simulink model "rls_param_est_2019_01_12"  (R2020a)
settings: Solver=VariableStepAuto  StartTime=0.0  StopTime=simlength  MaxStep=Ts  RelTol=Ts
undefined symbols (not defined in the file or in its folder): iniP11, iniP12, iniP13, iniP14, iniP21, iniP22, iniP23, iniP24, iniP31, iniP32, iniP33, iniP34, iniP41, iniP42, iniP43, iniP44, lambda, simlength, Tc, Tcontrol, Ts
libraries: cstblocks x5, simulink x1
settings Model: SimulationMode=accelerator  Creator=ltnbda  LastModifiedBy=dbagn
settings DataIOCC: ReturnWorkspaceOutputs=off
settings DebuggingCC: ArithmeticOperatorsInVariantConditions=warning
settings SFSimCC: CustomCodeUndefinedFunction=UseInterfaceOnly

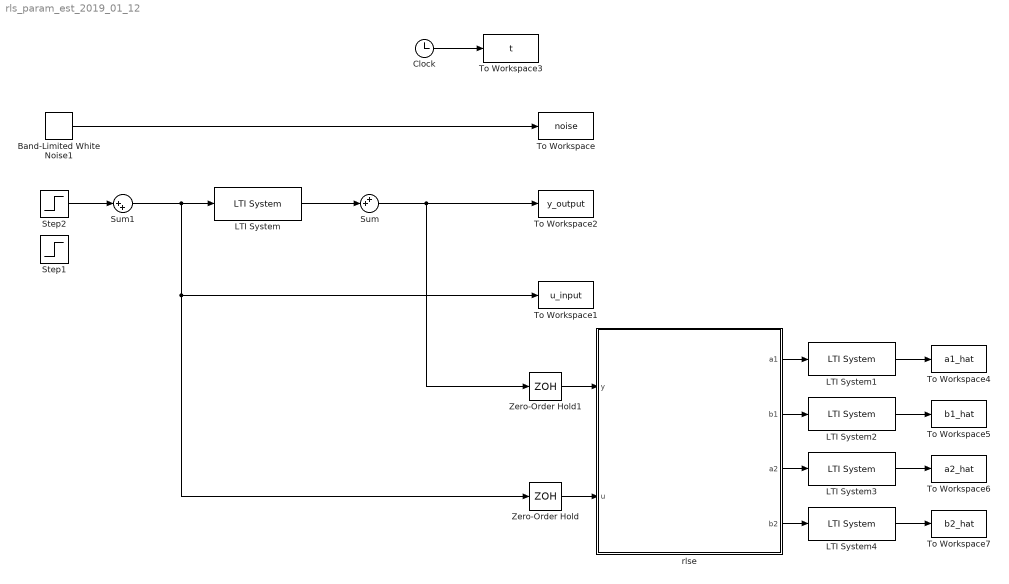
== system rls_param_est_2019_01_12 ==
  Band-Limited White Noise1 : simulink/Sources/Band-Limited White Noise  Cov=[1e-12]  Ts=Ts  seed=[0]
  Clock : Clock
  LTI System : cstblocks/LTI System  sys=sysIc  IC=[]
  LTI System{1..4} (4 alike) : cstblocks/LTI System  sys=filterd  IC=[]
  Step1 : Step  Time=simlength/2  After=0.5  SampleTime=Tcontrol
  Step2 : Step  Time=0.05  After=0.5  SampleTime=Tcontrol
  Sum : Sum  Inputs=++|
  Sum1 : Sum  Inputs=|++
  To Workspace : ToWorkspace  VariableName=noise  SampleTime=Tc
      settings: MaxDataPoints=Nc
  To Workspace1 : ToWorkspace  VariableName=u_input  SampleTime=Tc
      settings: MaxDataPoints=Nc
  To Workspace2 : ToWorkspace  VariableName=y_output  SampleTime=Tc
      settings: MaxDataPoints=Nc
  To Workspace3 : ToWorkspace  VariableName=t  SampleTime=Tc
      settings: MaxDataPoints=Nc
  To Workspace4 : ToWorkspace  VariableName=a1_hat  SampleTime=Tc
      settings: MaxDataPoints=Nc
  To Workspace5 : ToWorkspace  VariableName=b1_hat  SampleTime=Tc
      settings: MaxDataPoints=Nc
  To Workspace6 : ToWorkspace  VariableName=a2_hat  SampleTime=Tc
      settings: MaxDataPoints=Nc
  To Workspace7 : ToWorkspace  VariableName=b2_hat  SampleTime=Tc
      settings: MaxDataPoints=Nc
  Zero-Order Hold : ZeroOrderHold  SampleTime=Tcontrol
  Zero-Order Hold1 : ZeroOrderHold  SampleTime=Tcontrol
  rlse : Subsystem
  wires:
  LTI System/1 -> Sum/2
  Zero-Order Hold/1 -> rlse/2(u)
  Zero-Order Hold1/1 -> rlse/1(y)
  Sum/1 -> To Workspace2/1, Zero-Order Hold1/1
  Sum1/1 -> Zero-Order Hold/1, To Workspace1/1, LTI System/1
  Band-Limited White Noise1/1 -> To Workspace/1
  Clock/1 -> To Workspace3/1
  rlse/1(a1) -> LTI System1/1
  rlse/3(a2) -> LTI System3/1
  rlse/4(b2) -> LTI System4/1
  rlse/2(b1) -> LTI System2/1
  LTI System1/1 -> To Workspace4/1
  LTI System2/1 -> To Workspace5/1
  LTI System3/1 -> To Workspace6/1
  LTI System4/1 -> To Workspace7/1
  Step2/1 -> Sum1/1

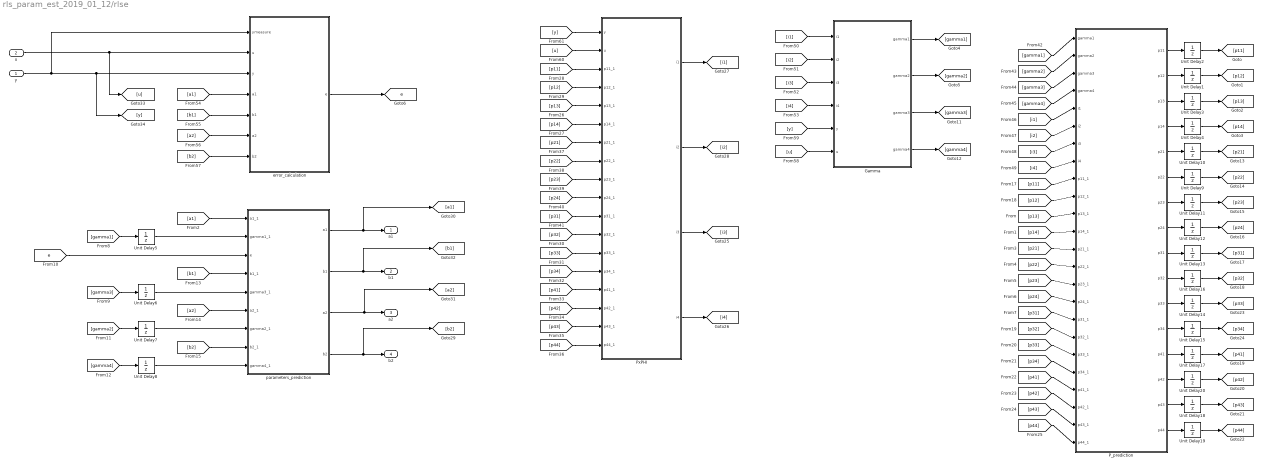
== system rls_param_est_2019_01_12/rlse ==
  y : Inport
  u : Inport  Port=2
  Gamma : Subsystem
  P_prediction : Subsystem
  PxPHI : Subsystem
  Unit Delay1 : UnitDelay  InitialCondition=iniP12  SampleTime=Tcontrol  HasFrameUpgradeWarning=on
  Unit Delay10 : UnitDelay  InitialCondition=iniP21  SampleTime=Tcontrol  HasFrameUpgradeWarning=on
  Unit Delay11 : UnitDelay  InitialCondition=iniP23  SampleTime=Tcontrol  HasFrameUpgradeWarning=on
  Unit Delay12 : UnitDelay  InitialCondition=iniP24  SampleTime=Tcontrol  HasFrameUpgradeWarning=on
  Unit Delay13 : UnitDelay  InitialCondition=iniP31  SampleTime=Tcontrol  HasFrameUpgradeWarning=on
  Unit Delay14 : UnitDelay  InitialCondition=iniP33  SampleTime=Tcontrol  HasFrameUpgradeWarning=on
  Unit Delay15 : UnitDelay  InitialCondition=iniP34  SampleTime=Tcontrol  HasFrameUpgradeWarning=on
  Unit Delay16 : UnitDelay  InitialCondition=iniP32  SampleTime=Tcontrol  HasFrameUpgradeWarning=on
  Unit Delay17 : UnitDelay  InitialCondition=iniP41  SampleTime=Tcontrol  HasFrameUpgradeWarning=on
  Unit Delay18 : UnitDelay  InitialCondition=iniP43  SampleTime=Tcontrol  HasFrameUpgradeWarning=on
  Unit Delay19 : UnitDelay  InitialCondition=iniP44  SampleTime=Tcontrol  HasFrameUpgradeWarning=on
  Unit Delay2 : UnitDelay  InitialCondition=iniP11  SampleTime=Tcontrol  HasFrameUpgradeWarning=on
  Unit Delay20 : UnitDelay  InitialCondition=iniP42  SampleTime=Tcontrol  HasFrameUpgradeWarning=on
  Unit Delay3 : UnitDelay  InitialCondition=iniP13  SampleTime=Tcontrol  HasFrameUpgradeWarning=on
  Unit Delay4 : UnitDelay  InitialCondition=iniP14  SampleTime=Tcontrol  HasFrameUpgradeWarning=on
  Unit Delay{5..8} (4 alike) : UnitDelay  SampleTime=Tcontrol  HasFrameUpgradeWarning=on
  Unit Delay9 : UnitDelay  InitialCondition=iniP22  SampleTime=Tcontrol  HasFrameUpgradeWarning=on
  error_calculation : Subsystem
  parameters_prediction : Subsystem
  a1 : Outport  VectorParamsAs1DForOutWhenUnconnected=off
  b1 : Outport  Port=2  VectorParamsAs1DForOutWhenUnconnected=off
  a2 : Outport  Port=3  VectorParamsAs1DForOutWhenUnconnected=off
  b2 : Outport  Port=4  VectorParamsAs1DForOutWhenUnconnected=off
  tag scope: e=global
  wires:
  u/1 -> [u], error_calculation/2(u)
  Unit Delay2/1 -> [p11]
  [gamma1] -> Unit Delay5/1
  [gamma3] -> Unit Delay6/1
  Unit Delay1/1 -> [p12]
  Unit Delay3/1 -> [p13]
  Unit Delay4/1 -> [p14]
  Unit Delay5/1 -> parameters_prediction/2(gamma1_1)
  Unit Delay6/1 -> parameters_prediction/5(gamma3_1)
  error_calculation/1(e) -> [e]
  [e] -> parameters_prediction/3(e)
  [gamma4] -> Unit Delay8/1
  [gamma2] -> Unit Delay7/1
  Unit Delay7/1 -> parameters_prediction/7(gamma2_1)
  Unit Delay8/1 -> parameters_prediction/9(gamma4_1)
  Gamma/1(gamma1) -> [gamma1]
  Gamma/2(gamma2) -> [gamma2]
  Gamma/3(gamma3) -> [gamma3]
  Gamma/4(gamma4) -> [gamma4]
  P_prediction/1(p11) -> Unit Delay2/1
  P_prediction/2(p12) -> Unit Delay1/1
  P_prediction/3(p13) -> Unit Delay3/1
  P_prediction/4(p14) -> Unit Delay4/1
  P_prediction/8(p24) -> Unit Delay12/1
  P_prediction/7(p23) -> Unit Delay11/1
  P_prediction/6(p22) -> Unit Delay9/1
  P_prediction/5(p21) -> Unit Delay10/1
  Unit Delay12/1 -> [p24]
  Unit Delay11/1 -> [p23]
  Unit Delay9/1 -> [p22]
  Unit Delay10/1 -> [p21]
  Unit Delay17/1 -> [p41]
  Unit Delay20/1 -> [p42]
  Unit Delay18/1 -> [p43]
  Unit Delay19/1 -> [p44]
  P_prediction/13(p41) -> Unit Delay17/1
  P_prediction/14(p42) -> Unit Delay20/1
  P_prediction/15(p43) -> Unit Delay18/1
  P_prediction/16(p44) -> Unit Delay19/1
  P_prediction/12(p34) -> Unit Delay15/1
  P_prediction/11(p33) -> Unit Delay14/1
  P_prediction/10(p32) -> Unit Delay16/1
  P_prediction/9(p31) -> Unit Delay13/1
  Unit Delay15/1 -> [p34]
  Unit Delay14/1 -> [p33]
  Unit Delay16/1 -> [p32]
  Unit Delay13/1 -> [p31]
  [p11] -> P_prediction/9(p11_1)
  [p13] -> P_prediction/11(p13_1)
  [p12] -> P_prediction/10(p12_1)
  [p14] -> P_prediction/12(p14_1)
  [p21] -> P_prediction/13(p21_1)
  [p22] -> P_prediction/14(p22_1)
  [p23] -> P_prediction/15(p23_1)
  [p24] -> P_prediction/16(p24_1)
  [p31] -> P_prediction/17(p31_1)
  [p32] -> P_prediction/18(p32_1)
  [p33] -> P_prediction/19(p33_1)
  [p34] -> P_prediction/20(p34_1)
  [p41] -> P_prediction/21(p41_1)
  [p42] -> P_prediction/22(p42_1)
  [p43] -> P_prediction/23(p43_1)
  [p44] -> P_prediction/24(p44_1)
  [p44] -> PxPHI/18(p44_1)
  [p43] -> PxPHI/17(p43_1)
  [p42] -> PxPHI/16(p42_1)
  [p41] -> PxPHI/15(p41_1)
  [p34] -> PxPHI/14(p34_1)
  [p33] -> PxPHI/13(p33_1)
  [p32] -> PxPHI/12(p32_1)
  [p31] -> PxPHI/11(p31_1)
  [p24] -> PxPHI/10(p24_1)
  [p23] -> PxPHI/9(p23_1)
  [p22] -> PxPHI/8(p22_1)
  [p21] -> PxPHI/7(p21_1)
  [p14] -> PxPHI/6(p14_1)
  [p12] -> PxPHI/4(p12_1)
  [p13] -> PxPHI/5(p13_1)
  [p11] -> PxPHI/3(p11_1)
  [gamma1] -> P_prediction/1(gamma1)
  [gamma2] -> P_prediction/2(gamma2)
  [gamma3] -> P_prediction/3(gamma3)
  [gamma4] -> P_prediction/4(gamma4)
  PxPHI/4(i4) -> [i4]
  PxPHI/3(i3) -> [i3]
  PxPHI/2(i2) -> [i2]
  PxPHI/1(i1) -> [i1]
  [i1] -> P_prediction/5(i1)
  [i2] -> P_prediction/6(i2)
  [i3] -> P_prediction/7(i3)
  [i4] -> P_prediction/8(i4)
  [i2] -> Gamma/2(i2)
  [i1] -> Gamma/1(i1)
  [i3] -> Gamma/3(i3)
  [i4] -> Gamma/4(i4)
  parameters_prediction/4(b2) -> [b2], b2/1
  parameters_prediction/3(a2) -> [a2], a2/1
  parameters_prediction/2(b1) -> [b1], b1/1
  parameters_prediction/1(a1) -> [a1], a1/1
  [a1] -> error_calculation/4(a1)
  [b1] -> error_calculation/5(b1)
  [a2] -> error_calculation/6(a2)
  [b2] -> error_calculation/7(b2)
  [u] -> Gamma/6(u)
  [y] -> Gamma/5(y)
  [y] -> PxPHI/1(y)
  [u] -> PxPHI/2(u)
  y/1 -> [y], error_calculation/3(y), error_calculation/1(ymeasure)
  [a1] -> parameters_prediction/1(a1_1)
  [b1] -> parameters_prediction/4(b1_1)
  [a2] -> parameters_prediction/6(a2_1)
  [b2] -> parameters_prediction/8(b2_1)

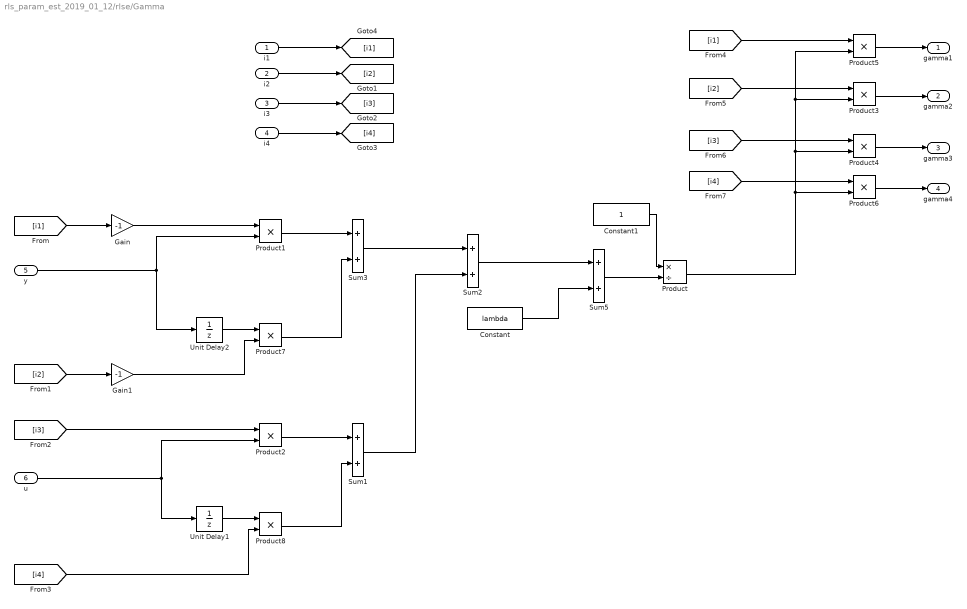
== system rls_param_est_2019_01_12/rlse/Gamma ==
  i1 : Inport
  i2 : Inport  Port=2
  i3 : Inport  Port=3
  i4 : Inport  Port=4
  y : Inport  Port=5
  u : Inport  Port=6
  Constant : Constant  Value=lambda
  Constant1 : Constant
  Gain : Gain  Gain=-1
  Gain1 : Gain  Gain=-1
  Product : Product  Inputs=*/
  Product{1..8} (8 alike) : Product
  Sum{1..3,5} (4 alike) : Sum
  Unit Delay1 : UnitDelay  SampleTime=Tcontrol  HasFrameUpgradeWarning=on
  Unit Delay2 : UnitDelay  SampleTime=Tcontrol  HasFrameUpgradeWarning=on
  gamma1 : Outport  VectorParamsAs1DForOutWhenUnconnected=off
  gamma2 : Outport  Port=2  VectorParamsAs1DForOutWhenUnconnected=off
  gamma3 : Outport  Port=3  VectorParamsAs1DForOutWhenUnconnected=off
  gamma4 : Outport  Port=4  VectorParamsAs1DForOutWhenUnconnected=off
  wires:
  u/1 -> Product2/2, Unit Delay1/1
  Gain/1 -> Product1/1
  y/1 -> Product1/2, Unit Delay2/1
  Constant1/1 -> Product/1
  Product3/1 -> gamma2/1
  Product5/1 -> gamma1/1
  Product4/1 -> gamma3/1
  Product6/1 -> gamma4/1
  Product1/1 -> Sum3/1
  Unit Delay2/1 -> Product7/1
  Gain1/1 -> Product7/2
  Product7/1 -> Sum3/2
  Product2/1 -> Sum1/1
  Product8/1 -> Sum1/2
  Sum3/1 -> Sum2/1
  Sum1/1 -> Sum2/2
  Product/1 -> Product6/2, Product4/2, Product3/2, Product5/2
  Sum2/1 -> Sum5/1
  Constant/1 -> Sum5/2
  Sum5/1 -> Product/2
  i1/1 -> [i1]
  i2/1 -> [i2]
  i3/1 -> [i3]
  i4/1 -> [i4]
  [i1] -> Gain/1
  [i2] -> Gain1/1
  [i3] -> Product2/1
  [i4] -> Product8/2
  [i1] -> Product5/1
  [i2] -> Product3/1
  [i3] -> Product4/1
  [i4] -> Product6/1
  Unit Delay1/1 -> Product8/1

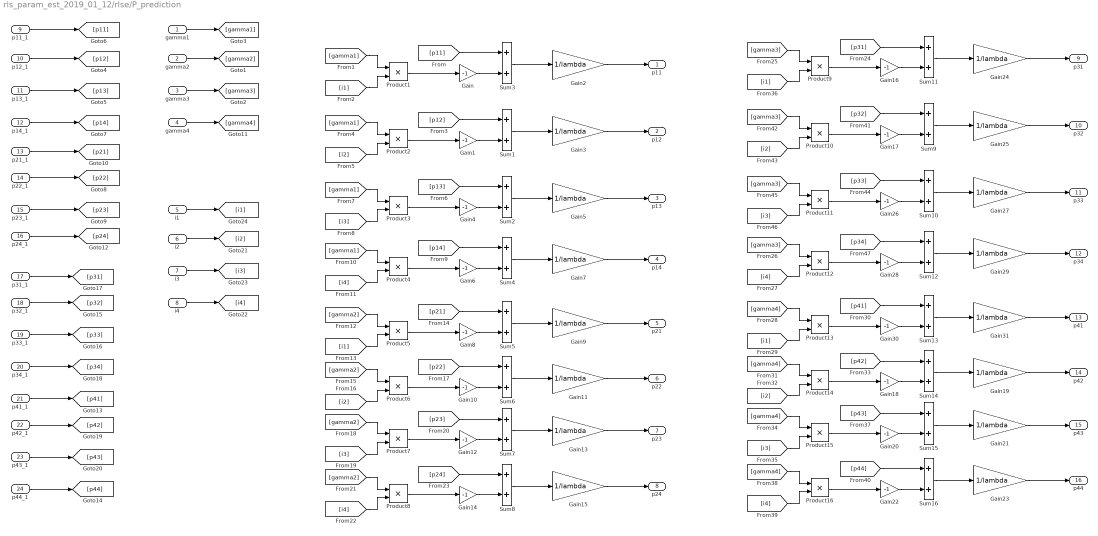
== system rls_param_est_2019_01_12/rlse/P_prediction ==
  gamma1 : Inport
  gamma2 : Inport  Port=2
  gamma3 : Inport  Port=3
  gamma4 : Inport  Port=4
  i1 : Inport  Port=5
  i2 : Inport  Port=6
  i3 : Inport  Port=7
  i4 : Inport  Port=8
  p11_1 : Inport  Port=9
  p12_1 : Inport  Port=10
  p13_1 : Inport  Port=11
  p14_1 : Inport  Port=12
  p21_1 : Inport  Port=13
  p22_1 : Inport  Port=14
  p23_1 : Inport  Port=15
  p24_1 : Inport  Port=16
  p31_1 : Inport  Port=17
  p32_1 : Inport  Port=18
  p33_1 : Inport  Port=19
  p34_1 : Inport  Port=20
  p41_1 : Inport  Port=21
  p42_1 : Inport  Port=22
  p43_1 : Inport  Port=23
  p44_1 : Inport  Port=24
  Gain{,1,4,6,8,10,12,14,16..18,20,22,26,28,30} (16 alike) : Gain  Gain=-1
  Gain{2..3,5,7,9,11,13,15,19,21,23..25,27,29,31} (16 alike) : Gain  Gain=1/lambda
  Product{1..16} (16 alike) : Product
  Sum{1..16} (16 alike) : Sum
  p11 : Outport  VectorParamsAs1DForOutWhenUnconnected=off
  p12 : Outport  Port=2  VectorParamsAs1DForOutWhenUnconnected=off
  p13 : Outport  Port=3  VectorParamsAs1DForOutWhenUnconnected=off
  p14 : Outport  Port=4  VectorParamsAs1DForOutWhenUnconnected=off
  p21 : Outport  Port=5  VectorParamsAs1DForOutWhenUnconnected=off
  p22 : Outport  Port=6  VectorParamsAs1DForOutWhenUnconnected=off
  p23 : Outport  Port=7  VectorParamsAs1DForOutWhenUnconnected=off
  p24 : Outport  Port=8  VectorParamsAs1DForOutWhenUnconnected=off
  p31 : Outport  Port=9  VectorParamsAs1DForOutWhenUnconnected=off
  p32 : Outport  Port=10  VectorParamsAs1DForOutWhenUnconnected=off
  p33 : Outport  Port=11  VectorParamsAs1DForOutWhenUnconnected=off
  p34 : Outport  Port=12  VectorParamsAs1DForOutWhenUnconnected=off
  p41 : Outport  Port=13  VectorParamsAs1DForOutWhenUnconnected=off
  p42 : Outport  Port=14  VectorParamsAs1DForOutWhenUnconnected=off
  p43 : Outport  Port=15  VectorParamsAs1DForOutWhenUnconnected=off
  p44 : Outport  Port=16  VectorParamsAs1DForOutWhenUnconnected=off
  wires:
  p11_1/1 -> [p11]
  p12_1/1 -> [p12]
  p13_1/1 -> [p13]
  p14_1/1 -> [p14]
  p21_1/1 -> [p21]
  p22_1/1 -> [p22]
  p23_1/1 -> [p23]
  p24_1/1 -> [p24]
  p31_1/1 -> [p31]
  p32_1/1 -> [p32]
  p33_1/1 -> [p33]
  p34_1/1 -> [p34]
  p41_1/1 -> [p41]
  p42_1/1 -> [p42]
  p43_1/1 -> [p43]
  p44_1/1 -> [p44]
  gamma1/1 -> [gamma1]
  gamma3/1 -> [gamma3]
  gamma2/1 -> [gamma2]
  gamma4/1 -> [gamma4]
  i4/1 -> [i4]
  i2/1 -> [i2]
  i3/1 -> [i3]
  i1/1 -> [i1]
  [p11] -> Sum3/1
  Gain/1 -> Sum3/2
  Product1/1 -> Gain/1
  [gamma1] -> Product1/1
  [i1] -> Product1/2
  Sum3/1 -> Gain2/1
  Gain2/1 -> p11/1
  Sum1/1 -> Gain3/1
  [i2] -> Product2/2
  [gamma1] -> Product2/1
  Product2/1 -> Gain1/1
  Gain1/1 -> Sum1/2
  [p12] -> Sum1/1
  Gain3/1 -> p12/1
  Gain5/1 -> p13/1
  [p13] -> Sum2/1
  Gain4/1 -> Sum2/2
  Product3/1 -> Gain4/1
  [gamma1] -> Product3/1
  [i3] -> Product3/2
  Sum2/1 -> Gain5/1
  Sum4/1 -> Gain7/1
  [i4] -> Product4/2
  [gamma1] -> Product4/1
  Product4/1 -> Gain6/1
  Gain6/1 -> Sum4/2
  [p14] -> Sum4/1
  Gain7/1 -> p14/1
  Gain9/1 -> p21/1
  [p21] -> Sum5/1
  Gain8/1 -> Sum5/2
  Product5/1 -> Gain8/1
  [gamma2] -> Product5/1
  [i1] -> Product5/2
  Sum5/1 -> Gain9/1
  Sum6/1 -> Gain11/1
  [i2] -> Product6/2
  [gamma2] -> Product6/1
  Product6/1 -> Gain10/1
  Gain10/1 -> Sum6/2
  [p22] -> Sum6/1
  Gain11/1 -> p22/1
  Gain13/1 -> p23/1
  [p23] -> Sum7/1
  Gain12/1 -> Sum7/2
  Product7/1 -> Gain12/1
  [gamma2] -> Product7/1
  [i3] -> Product7/2
  Sum7/1 -> Gain13/1
  Sum8/1 -> Gain15/1
  [i4] -> Product8/2
  [gamma2] -> Product8/1
  Product8/1 -> Gain14/1
  Gain14/1 -> Sum8/2
  [p24] -> Sum8/1
  Gain15/1 -> p24/1
  Gain23/1 -> p44/1
  [p44] -> Sum16/1
  Gain22/1 -> Sum16/2
  Product16/1 -> Gain22/1
  [gamma4] -> Product16/1
  [i4] -> Product16/2
  Sum16/1 -> Gain23/1
  Sum15/1 -> Gain21/1
  [i3] -> Product15/2
  [gamma4] -> Product15/1
  Product15/1 -> Gain20/1
  Gain20/1 -> Sum15/2
  [p43] -> Sum15/1
  Gain21/1 -> p43/1
  Gain19/1 -> p42/1
  [p42] -> Sum14/1
  Gain18/1 -> Sum14/2
  Product14/1 -> Gain18/1
  [gamma4] -> Product14/1
  [i2] -> Product14/2
  Sum14/1 -> Gain19/1
  Sum13/1 -> Gain31/1
  [i1] -> Product13/2
  [gamma4] -> Product13/1
  Product13/1 -> Gain30/1
  Gain30/1 -> Sum13/2
  [p41] -> Sum13/1
  Gain31/1 -> p41/1
  Gain29/1 -> p34/1
  [p34] -> Sum12/1
  Gain28/1 -> Sum12/2
  Product12/1 -> Gain28/1
  [gamma3] -> Product12/1
  [i4] -> Product12/2
  Sum12/1 -> Gain29/1
  Sum10/1 -> Gain27/1
  [i3] -> Product11/2
  [gamma3] -> Product11/1
  Product11/1 -> Gain26/1
  Gain26/1 -> Sum10/2
  [p33] -> Sum10/1
  Gain27/1 -> p33/1
  Gain25/1 -> p32/1
  [p32] -> Sum9/1
  Gain17/1 -> Sum9/2
  Product10/1 -> Gain17/1
  [gamma3] -> Product10/1
  [i2] -> Product10/2
  Sum9/1 -> Gain25/1
  Gain24/1 -> p31/1
  Sum11/1 -> Gain24/1
  [i1] -> Product9/2
  [gamma3] -> Product9/1
  Product9/1 -> Gain16/1
  Gain16/1 -> Sum11/2
  [p31] -> Sum11/1

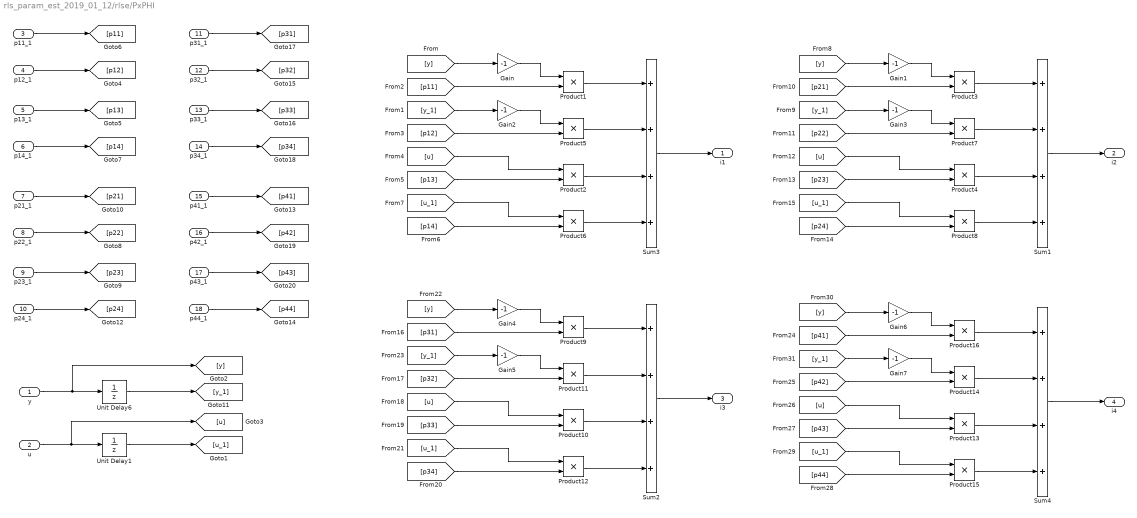
== system rls_param_est_2019_01_12/rlse/PxPHI ==
  y : Inport
  u : Inport  Port=2
  p11_1 : Inport  Port=3
  p12_1 : Inport  Port=4
  p13_1 : Inport  Port=5
  p14_1 : Inport  Port=6
  p21_1 : Inport  Port=7
  p22_1 : Inport  Port=8
  p23_1 : Inport  Port=9
  p24_1 : Inport  Port=10
  p31_1 : Inport  Port=11
  p32_1 : Inport  Port=12
  p33_1 : Inport  Port=13
  p34_1 : Inport  Port=14
  p41_1 : Inport  Port=15
  p42_1 : Inport  Port=16
  p43_1 : Inport  Port=17
  p44_1 : Inport  Port=18
  Gain{,1..7} (8 alike) : Gain  Gain=-1
  Product{1..16} (16 alike) : Product
  Sum{1..4} (4 alike) : Sum  Inputs=++++
  Unit Delay1 : UnitDelay  SampleTime=Tcontrol  HasFrameUpgradeWarning=on
  Unit Delay6 : UnitDelay  SampleTime=Tcontrol  HasFrameUpgradeWarning=on
  i1 : Outport  VectorParamsAs1DForOutWhenUnconnected=off
  i2 : Outport  Port=2  VectorParamsAs1DForOutWhenUnconnected=off
  i3 : Outport  Port=3  VectorParamsAs1DForOutWhenUnconnected=off
  i4 : Outport  Port=4  VectorParamsAs1DForOutWhenUnconnected=off
  wires:
  Sum3/1 -> i1/1
  Product1/1 -> Sum3/1
  Unit Delay6/1 -> [y_1]
  y/1 -> [y], Unit Delay6/1
  u/1 -> [u], Unit Delay1/1
  Unit Delay1/1 -> [u_1]
  p12_1/1 -> [p12]
  p13_1/1 -> [p13]
  p11_1/1 -> [p11]
  p14_1/1 -> [p14]
  p22_1/1 -> [p22]
  p21_1/1 -> [p21]
  p23_1/1 -> [p23]
  p24_1/1 -> [p24]
  p31_1/1 -> [p31]
  p32_1/1 -> [p32]
  p33_1/1 -> [p33]
  p34_1/1 -> [p34]
  p41_1/1 -> [p41]
  p42_1/1 -> [p42]
  p43_1/1 -> [p43]
  p44_1/1 -> [p44]
  Gain/1 -> Product1/1
  Gain2/1 -> Product5/1
  Product5/1 -> Sum3/2
  Product2/1 -> Sum3/3
  Product6/1 -> Sum3/4
  [y] -> Gain/1
  [y_1] -> Gain2/1
  [p11] -> Product1/2
  [p12] -> Product5/2
  [u] -> Product2/1
  [p13] -> Product2/2
  [p14] -> Product6/2
  [u_1] -> Product6/1
  [u_1] -> Product8/1
  [p24] -> Product8/2
  [p23] -> Product4/2
  [u] -> Product4/1
  [p22] -> Product7/2
  [p21] -> Product3/2
  [y_1] -> Gain3/1
  [y] -> Gain1/1
  Product8/1 -> Sum1/4
  Product4/1 -> Sum1/3
  Product7/1 -> Sum1/2
  Gain3/1 -> Product7/1
  Gain1/1 -> Product3/1
  Product3/1 -> Sum1/1
  Sum1/1 -> i2/1
  Sum2/1 -> i3/1
  Product9/1 -> Sum2/1
  Gain4/1 -> Product9/1
  Gain5/1 -> Product11/1
  Product11/1 -> Sum2/2
  Product10/1 -> Sum2/3
  Product12/1 -> Sum2/4
  [y] -> Gain4/1
  [y_1] -> Gain5/1
  [p31] -> Product9/2
  [p32] -> Product11/2
  [u] -> Product10/1
  [p33] -> Product10/2
  [p34] -> Product12/2
  [u_1] -> Product12/1
  [u_1] -> Product15/1
  [p44] -> Product15/2
  [p43] -> Product13/2
  [u] -> Product13/1
  [p42] -> Product14/2
  [p41] -> Product16/2
  [y_1] -> Gain7/1
  [y] -> Gain6/1
  Product15/1 -> Sum4/4
  Product13/1 -> Sum4/3
  Product14/1 -> Sum4/2
  Gain7/1 -> Product14/1
  Gain6/1 -> Product16/1
  Product16/1 -> Sum4/1
  Sum4/1 -> i4/1

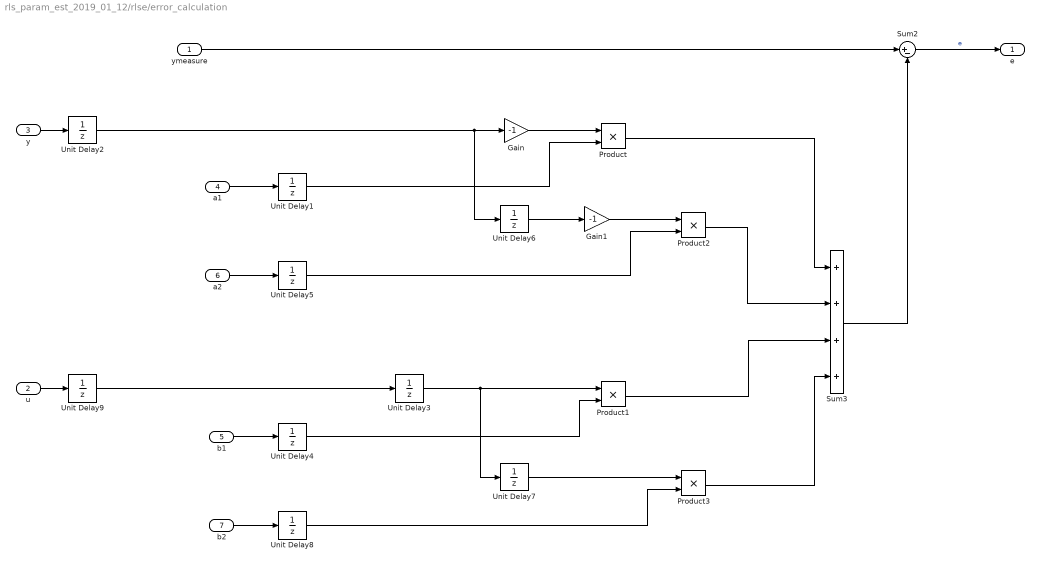
== system rls_param_est_2019_01_12/rlse/error_calculation ==
  ymeasure : Inport
  u : Inport  Port=2
  y : Inport  Port=3
  a1 : Inport  Port=4
  b1 : Inport  Port=5
  a2 : Inport  Port=6
  b2 : Inport  Port=7
  Gain : Gain  Gain=-1
  Gain1 : Gain  Gain=-1
  Product{,1..3} (4 alike) : Product
  Sum2 : Sum  Inputs=|+-
  Sum3 : Sum  Inputs=++++
  Unit Delay{1..9} (9 alike) : UnitDelay  SampleTime=Tcontrol  HasFrameUpgradeWarning=on
  e : Outport  VectorParamsAs1DForOutWhenUnconnected=off
  wires:
  Gain/1 -> Product/1
  Sum3/1 -> Sum2/2
  Sum2/1 -> e/1  "e"
  a1/1 -> Unit Delay1/1
  b1/1 -> Unit Delay4/1
  y/1 -> Unit Delay2/1
  Unit Delay1/1 -> Product/2
  Unit Delay3/1 -> Unit Delay7/1, Product1/1
  Unit Delay4/1 -> Product1/2
  Unit Delay5/1 -> Product2/2
  Unit Delay6/1 -> Gain1/1
  a2/1 -> Unit Delay5/1
  Gain1/1 -> Product2/1
  Product/1 -> Sum3/1
  Product2/1 -> Sum3/2
  Unit Delay8/1 -> Product3/2
  Unit Delay7/1 -> Product3/1
  b2/1 -> Unit Delay8/1
  Product1/1 -> Sum3/3
  Product3/1 -> Sum3/4
  ymeasure/1 -> Sum2/1
  u/1 -> Unit Delay9/1
  Unit Delay2/1 -> Unit Delay6/1, Gain/1
  Unit Delay9/1 -> Unit Delay3/1

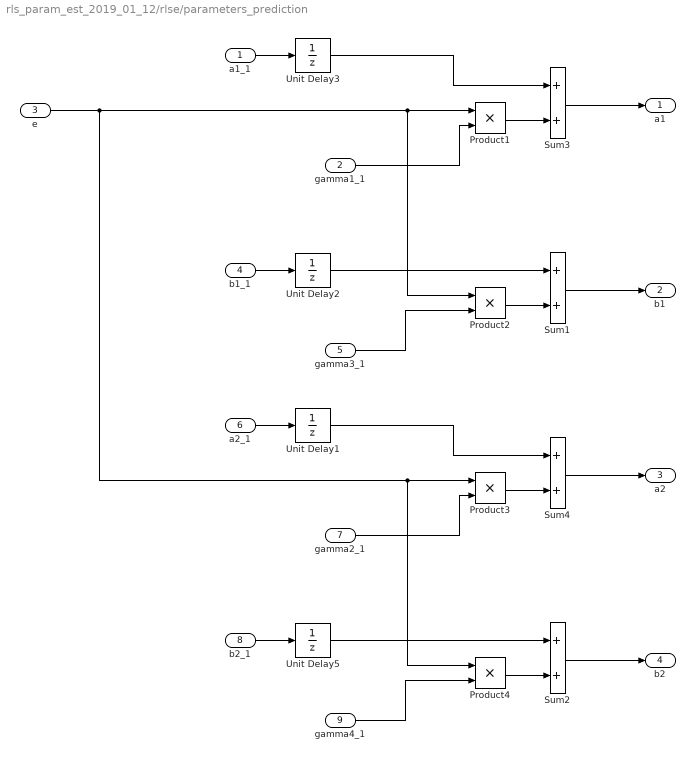
== system rls_param_est_2019_01_12/rlse/parameters_prediction ==
  a1_1 : Inport
  gamma1_1 : Inport  Port=2
  e : Inport  Port=3
  b1_1 : Inport  Port=4
  gamma3_1 : Inport  Port=5
  a2_1 : Inport  Port=6
  gamma2_1 : Inport  Port=7
  b2_1 : Inport  Port=8
  gamma4_1 : Inport  Port=9
  Product{1..4} (4 alike) : Product
  Sum{1..4} (4 alike) : Sum
  Unit Delay{1..3,5} (4 alike) : UnitDelay  SampleTime=Tcontrol  HasFrameUpgradeWarning=on
  a1 : Outport  VectorParamsAs1DForOutWhenUnconnected=off
  b1 : Outport  Port=2  VectorParamsAs1DForOutWhenUnconnected=off
  a2 : Outport  Port=3  VectorParamsAs1DForOutWhenUnconnected=off
  b2 : Outport  Port=4  VectorParamsAs1DForOutWhenUnconnected=off
  wires:
  gamma1_1/1 -> Product1/2
  Product1/1 -> Sum3/2
  Sum3/1 -> a1/1
  a1_1/1 -> Unit Delay3/1
  b1_1/1 -> Unit Delay2/1
  Sum1/1 -> b1/1
  Product2/1 -> Sum1/2
  gamma3_1/1 -> Product2/2
  gamma4_1/1 -> Product4/2
  Product4/1 -> Sum2/2
  Sum2/1 -> b2/1
  b2_1/1 -> Unit Delay5/1
  a2_1/1 -> Unit Delay1/1
  Sum4/1 -> a2/1
  Product3/1 -> Sum4/2
  e/1 -> Product3/1, Product4/1, Product2/1, Product1/1
  gamma2_1/1 -> Product3/2
  Unit Delay5/1 -> Sum2/1
  Unit Delay1/1 -> Sum4/1
  Unit Delay2/1 -> Sum1/1
  Unit Delay3/1 -> Sum3/1
